simulink model "flexibleBeamILCBF"  (R2021a)
settings: Solver=ode23t  StartTime=0.0  StopTime=Tend  FixedStep=Ts  RelTol=1e-2
values from neighbouring files (symbols this model uses):
  G = ss(ModelFlexiblePlateFirstPrinciple(POI,grids,a,b))    [ILCBF.m]    (also in ModelFlexiblePlateFirstPrinciple.m = G+(Cm(:,r)*Bm(r,:))/(s^2+2*zeta(r-1)*wn(r-1)*s+wn(r-1)^2))
  Ts = 1e-3    (= 0.001)    [GPSnapFlexiblePlate.m]
undefined symbols (not defined in the file or in its folder): x0x, x0y
libraries: dspsrcs4 x2, simulink x1
settings Model: Creator=s152009  LastModifiedBy=s152009

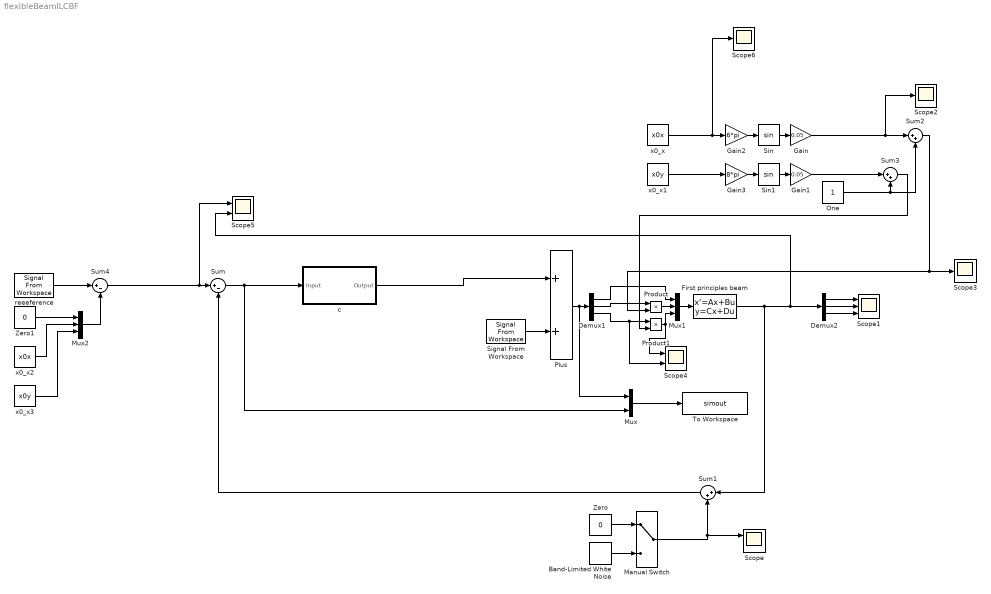
== system flexibleBeamILCBF ==
  Band-Limited White Noise : simulink/Sources/Band-Limited White Noise  Cov=[1e-16]  Ts=Ts  seed=[23341]
  Demux1 : Demux  Outputs=3
  Demux2 : Demux  Outputs=3
  First principles beam : StateSpace  A=G.A  B=G.B  C=G.C  D=G.D  InitialCondition=0
  Gain : Gain  Gain=0.05
  Gain1 : Gain  Gain=0.05
  Gain2 : Gain  Gain=6*pi
  Gain3 : Gain  Gain=8*pi
  Manual Switch : ManualSwitch
  Mux : Mux  Inputs=2
  Mux1 : Mux  Inputs=3
  Mux2 : Mux  Inputs=3
  One : Constant  OutDataTypeStr=Inherit: Inherit via back propagation
  Plus : Sum
  Product : Product
  Product1 : Product
  Scope : Scope  NumInputPorts=2
  Scope1 : Scope  NumInputPorts=3
  Scope2 : Scope
  Scope3 : Scope
  Scope4 : Scope  NumInputPorts=2
  Scope5 : Scope  NumInputPorts=2
  Scope6 : Scope
  Signal From Workspace : dspsrcs4/Signal From Workspace  X=f_j  Ts=Ts  nsamps=1  OutputAfterFinalValue=Setting to zero  ignoreOrWarnInputAndFrameLengths=off  OutputFrames=off
  Sin : Trigonometry
  Sin1 : Trigonometry
  Sum : Sum  Inputs=|+-
  Sum1 : Sum  Inputs=|++
  Sum2 : Sum  Inputs=|++
  Sum3 : Sum  Inputs=|++
  Sum4 : Sum  Inputs=|+-
  To Workspace : ToWorkspace  VariableName=simout  SampleTime=Ts
      settings: Save2DSignal=2-D array (concatenate along first dimension)
  Zero : Constant  Value=0  OutDataTypeStr=Inherit: Inherit via back propagation
  Zero1 : Constant  Value=0  OutDataTypeStr=Inherit: Inherit via back propagation
  c : Subsystem
  reeeference : dspsrcs4/Signal From Workspace  X=r  Ts=Ts  nsamps=1  OutputAfterFinalValue=Holding final value  ignoreOrWarnInputAndFrameLengths=off  OutputFrames=off
  x0_x : Constant  Value=x0x  SampleTime=0
  x0_x1 : Constant  Value=x0y  SampleTime=0
  x0_x2 : Constant  Value=x0x  SampleTime=0
  x0_x3 : Constant  Value=x0y  SampleTime=0
  wires:
  reeeference/1 -> Sum4/1
  Signal From Workspace/1 -> Plus/2
  Plus/1 -> Demux1/1, Mux/1
  Sum/1 -> c/1(Input), Mux/2
  Mux/1 -> To Workspace/1
  c/1(Output) -> Plus/1
  Sum1/1 -> Sum/2
  Manual Switch/1 -> Scope/1, Sum1/2
  Zero/1 -> Manual Switch/1
  Band-Limited White Noise/1 -> Manual Switch/2
  First principles beam/1 -> Scope5/2, Demux2/1, Sum1/1
  One/1 -> Sum2/2, Sum3/2
  Sin/1 -> Gain/1
  Gain/1 -> Scope2/1, Sum2/1
  Sin1/1 -> Gain1/1
  Gain1/1 -> Sum3/1
  Mux1/1 -> First principles beam/1
  Demux1/1 -> Mux1/1
  Product/1 -> Mux1/2
  Product1/1 -> Scope4/1, Mux1/3
  Demux1/2 -> Product/1
  Demux1/3 -> Scope4/2, Product1/1
  Sum2/1 -> Product/2, Scope3/1
  Sum3/1 -> Product1/2
  Demux2/1 -> Scope1/1
  Demux2/2 -> Scope1/2
  Demux2/3 -> Scope1/3
  Gain2/1 -> Sin/1
  Gain3/1 -> Sin1/1
  x0_x1/1 -> Gain3/1
  x0_x/1 -> Scope6/1, Gain2/1
  Sum4/1 -> Scope5/1, Sum/1
  Mux2/1 -> Sum4/2
  x0_x2/1 -> Mux2/2
  x0_x3/1 -> Mux2/3
  Zero1/1 -> Mux2/1

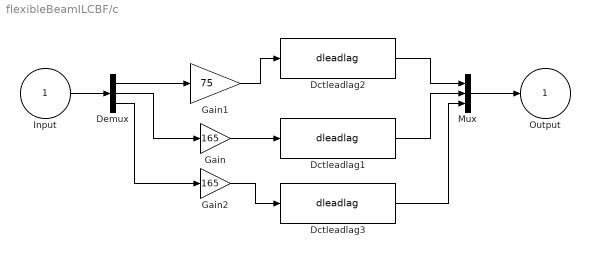
== system flexibleBeamILCBF/c ==
  Input : Inport
  Dctleadlag1 : S-Function  FunctionName=dleadlag  Parameters=f_num, f_den, 0.001  SFunctionDeploymentMode=off  EnableBusSupport=off  mask(dctools){f_num=1, f_den=10}
      mask prompts: f_num "Zero [Hz]"; f_den "Pole [Hz]"
      mask help: This block implements a discrete time leadlag filter.
      mask Display: disp('DCT leadlag')
  Dctleadlag2 : S-Function  FunctionName=dleadlag  Parameters=f_num, f_den, 0.001  SFunctionDeploymentMode=off  EnableBusSupport=off  mask(dctools){f_num=0.5, f_den=5}
      mask prompts: f_num "Zero [Hz]"; f_den "Pole [Hz]"
      mask help: This block implements a discrete time leadlag filter.
      mask Display: disp('DCT leadlag')
  Dctleadlag3 : S-Function  FunctionName=dleadlag  Parameters=f_num, f_den, 0.001  SFunctionDeploymentMode=off  EnableBusSupport=off  mask(dctools){f_num=1, f_den=10}
      mask prompts: f_num "Zero [Hz]"; f_den "Pole [Hz]"
      mask help: This block implements a discrete time leadlag filter.
      mask Display: disp('DCT leadlag')
  Demux : Demux  Outputs=3
  Gain : Gain  Gain=165
  Gain1 : Gain  Gain=75
  Gain2 : Gain  Gain=165
  Mux : Mux  Inputs=3
  Output : Outport
  wires:
  Gain1/1 -> Dctleadlag2/1
  Input/1 -> Demux/1
  Demux/1 -> Gain1/1
  Dctleadlag2/1 -> Mux/1
  Mux/1 -> Output/1
  Demux/2 -> Gain/1
  Demux/3 -> Gain2/1
  Gain/1 -> Dctleadlag1/1
  Gain2/1 -> Dctleadlag3/1
  Dctleadlag1/1 -> Mux/2
  Dctleadlag3/1 -> Mux/3
